simulink model "lqr_test"  (R2017a)
settings: Solver=ode4  StartTime=0.0  StopTime=5  FixedStep=Ts  RelTol=1e-3  EnableMultiTasking=on
values from neighbouring files (symbols this model uses):
  Ac = [0  1  0  0  0  0 ... (first row only)    [lqr_inner_synthesis.m]
  Bc = [0   0   0 ... (first row only)    [lqr_inner_synthesis.m]
  Cc = [1 0 0 0 0 0 ... (first row only)    [lqr_inner_synthesis.m]
  Ki_lqr = [8.66025403784  0  0; 0  0.1  0; 0  0  0.1]    [K_lqr.mat]    (also in lqr_inner_synthesis.m = -K(:,7:end))
  Kx_lqr = [13.6588017709 0 0 7.88446073405 0 0 0 0.182798226623 0 0 0 0.193348614018 ... (18 elements, 3x6)]    [K_lqr.mat]    (also in lqr_inner_synthesis.m = K(:,1:6))
undefined symbols (not defined in the file or in its folder): B_inner_inv, gra, KT, mass
settings Model: Creator=dtnguyen  LastModifiedBy=ducnguyen
settings DataIOCC: LimitDataPoints=on  SaveFormat=Array
settings OptimizationCC: DefaultParameterBehavior=Inlined  UseFloatMulNetSlope=on  InlineInvariantSignals=on  EfficientFloat2IntCast=on  LifeSpan=inf
settings DebuggingCC: SFUnexpectedBacktrackingDiag=warning  SFNoUnconditionalDefaultTransitionDiag=warning  SFExecutionAtInitializationDiag=none
settings HardwareCC: ProdBitPerPointer=32  ProdBitPerSizeT=32  ProdBitPerPtrDiffT=32  ProdLargestAtomicFloat=None  ProdIntDivRoundTo=Undefined  ProdEndianess=Unspecified  ProdWordSize=32  ProdHWDeviceType=32-bit Generic
settings ModelReferenceCC: PropagateSignalLabelsOutOfModel=off
settings RTWCC: GenerateReport=on  Toolchain=Catkin  BuildConfiguration=Faster Runs  LaunchReport=on  TargetLang=C++  CheckMdlBeforeBuild=Warning
settings GRTTargetCC: TargetLangStandard=C++03 (ISO)  GeneratePreprocessorConditionals=Disable all  MatFileLogging=off  MultiInstanceERTCode=on  CodeInterfacePackaging=C++ class  SupportNonFinite=off
settings ConfigComp: CovMetricSettings=dw  CovHtmlReporting=on  CovSaveCumulativeToWorkspaceVar=on  CovSaveSingleToWorkspaceVar=on  CovExternalEMLEnable=off

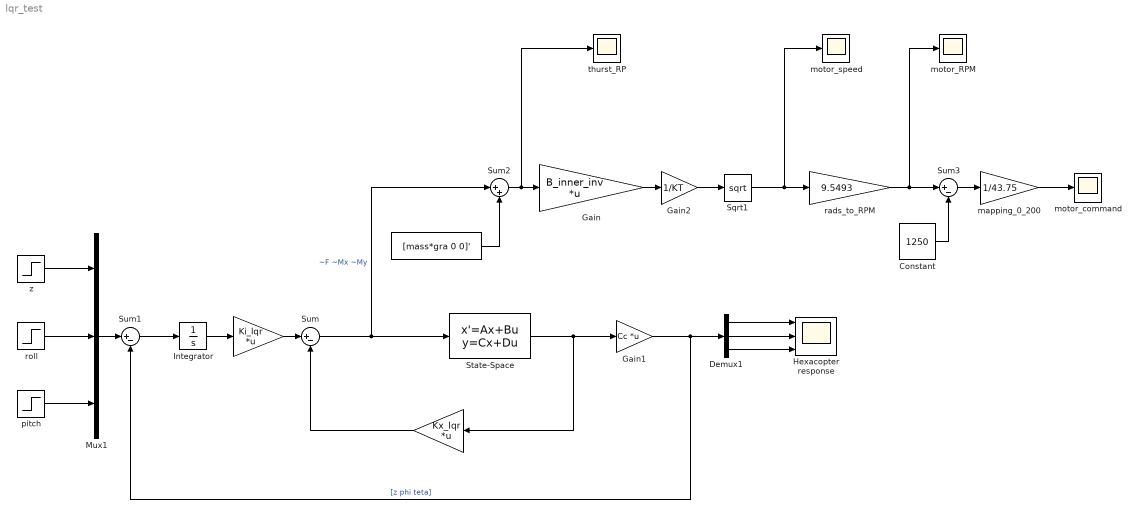
== system lqr_test ==
  " " : Gain  Gain=Ki_lqr  Multiplication=Matrix(K*u)
  "              " : Constant  Value=[mass*gra 0 0]'
  "                   " : Gain  Gain=Kx_lqr  Multiplication=Matrix(K*u)
  Constant : Constant  Value=1250  VectorParams1D=off  SampleTime=-1
  Demux1 : Demux  Outputs=3
  Gain : Gain  Gain=B_inner_inv  Multiplication=Matrix(K*u)
  Gain1 : Gain  Gain=Cc  Multiplication=Matrix(K*u)
  Gain2 : Gain  Gain=1/KT
  Hexacopter response : Scope  NumInputPorts=3
  Integrator : Integrator  InitialCondition=[0 0 0]
  Mux1 : Mux  Inputs=3
  Sqrt1 : Sqrt  SaturateOnIntegerOverflow=on
  State-Space : StateSpace  A=Ac  B=Bc  C=eye(6)  D=zeros(6,3)  X0=0
  Sum : Sum  Inputs=|+-
  Sum1 : Sum  Inputs=|+-
  Sum2 : Sum  Inputs=|++
  Sum3 : Sum  Inputs=|+-
  mapping_0_200 : Gain  Gain=1/43.75
  motor_RPM : Scope
  motor_command : Scope
  motor_speed : Scope
  pitch : Step  Time=0  After=-pi/18  SampleTime=0
  rads_to_RPM : Gain  Gain=9.5493
  roll : Step  Time=0  After=pi/18  SampleTime=0
  thurst_RP : Scope
  z : Step  Time=0  After=0.5  SampleTime=0
  wires:
  Sum/1 -> Sum2/1, State-Space/1  "~F ~Mx ~My"
  "                   "/1 -> Sum/2
  Integrator/1 -> " "/1
  " "/1 -> Sum/1
  Mux1/1 -> Sum1/1
  Demux1/2 -> Hexacopter response/2
  Demux1/1 -> Hexacopter response/1
  Demux1/3 -> Hexacopter response/3
  pitch/1 -> Mux1/3
  z/1 -> Mux1/1
  roll/1 -> Mux1/2
  Sum1/1 -> Integrator/1
  State-Space/1 -> Gain1/1, "                   "/1
  Gain1/1 -> Sum1/2, Demux1/1  "[z phi teta]"
  "              "/1 -> Sum2/2
  Sum2/1 -> thurst_RP/1, Gain/1
  Gain/1 -> Gain2/1
  Gain2/1 -> Sqrt1/1
  Sqrt1/1 -> rads_to_RPM/1, motor_speed/1
  rads_to_RPM/1 -> Sum3/1, motor_RPM/1
  mapping_0_200/1 -> motor_command/1
  Constant/1 -> Sum3/2
  Sum3/1 -> mapping_0_200/1
